simulink model "pressure_tank"  (R2017b)
settings: Solver=FixedStepAuto  StartTime=0.0  StopTime=100  FixedStep=0.01  RelTol=1e-3
libraries: simulink x1
settings Model: Creator=ernst  LastModifiedBy=ernst
settings DataIOCC: SaveFormat=StructureWithTime  SignalLogging=off  DSMLogging=off

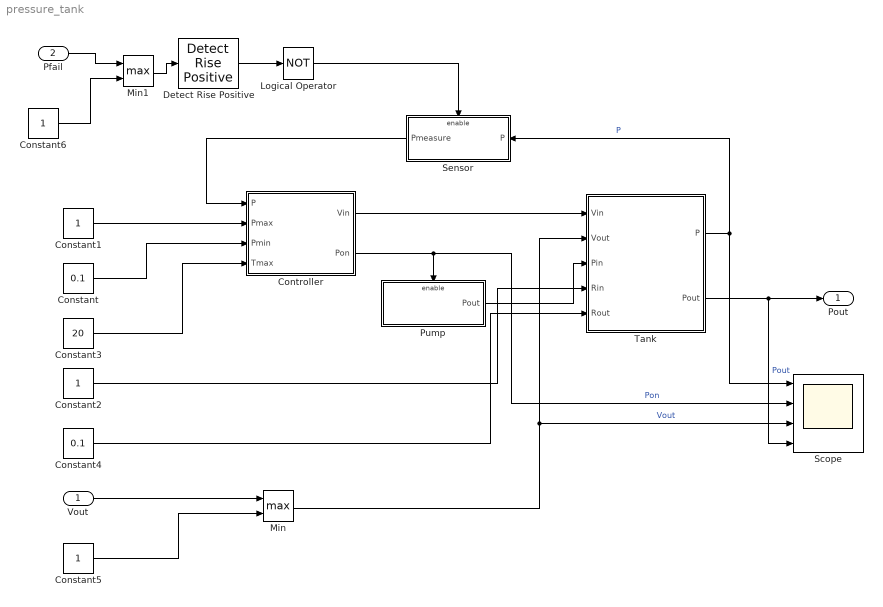
== system pressure_tank ==
  Vout : Inport
  Pfail : Inport  Port=2
  Constant : Constant  Value=0.1
  Constant{1..2,5..6} (4 alike) : Constant
  Constant3 : Constant  Value=20
  Constant4 : Constant  Value=0.1
  Controller : Stateflow chart  TreatAsAtomicUnit=on
  Detect Rise Positive : simulink/Logic and Bit Operations/Detect Rise Positive  vinit=0  OutDataTypeStr=boolean
  Logical Operator : Logic  Operator=NOT  AllPortsSameDT=off  OutDataTypeStr=boolean
  Min : MinMax  Function=max  Inputs=2
  Min1 : MinMax  Function=max  Inputs=2
  Pump : Subsystem
  Scope : Scope  NumInputPorts=4
  Sensor : Subsystem
  Tank : Subsystem
  Pout : Outport
  wires:
  Pump/1(Pout) -> Tank/3(Pin)
  Controller/1(Vin) -> Tank/1(Vin)
  Vout/1 -> Min/1
  Controller/2(Pon) -> Pump/Enable, Scope/2  "Pon"
  Tank/2(Pout) -> Pout/1, Scope/4  "Pout"
  Constant1/1 -> Controller/2(Pmax)
  Constant/1 -> Controller/3(Pmin)
  Tank/1("P ") -> Scope/1, Sensor/1(P)  "P"
  Sensor/1(Pmeasure) -> Controller/1(P)
  Min1/1 -> Detect Rise Positive/1
  Logical Operator/1 -> Sensor/Enable
  Constant2/1 -> Tank/4(Rin)
  Constant3/1 -> Controller/4(Tmax)
  Min/1 -> Tank/2(Vout), Scope/3  "Vout"
  Constant5/1 -> Min/2
  Constant4/1 -> Tank/5(Rout)
  Detect Rise Positive/1 -> Logical Operator/1
  Pfail/1 -> Min1/1
  Constant6/1 -> Min1/2

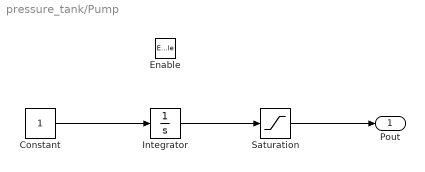
== system pressure_tank/Pump ==
  Enable : EnablePort
  Constant : Constant
  Integrator : Integrator
  Saturation : Saturate  UpperLimit=1  LowerLimit=0
  Pout : Outport
  wires:
  Integrator/1 -> Saturation/1
  Saturation/1 -> Pout/1
  Constant/1 -> Integrator/1

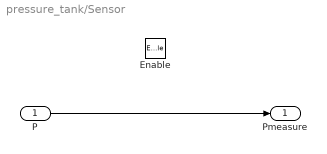
== system pressure_tank/Sensor ==
  P : Inport
  Enable : EnablePort
  Pmeasure : Outport
  wires:
  P/1 -> Pmeasure/1

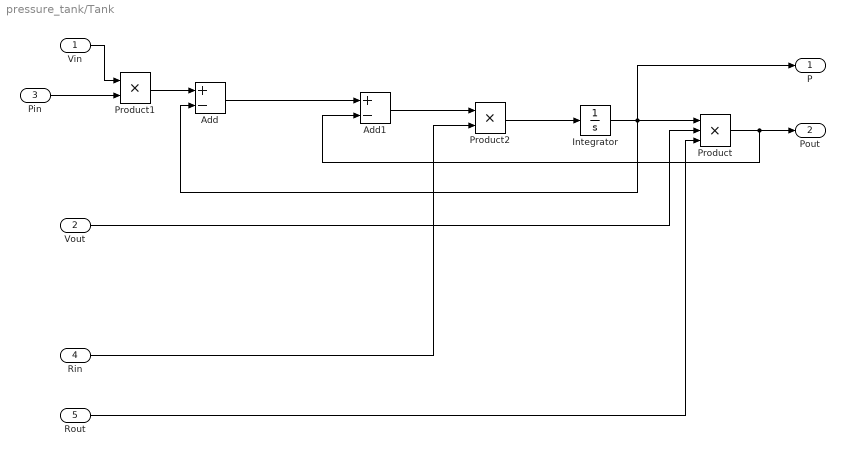
== system pressure_tank/Tank ==
  Vin : Inport
  Vout : Inport  Port=2
  Pin : Inport  Port=3
  Rin : Inport  Port=4
  Rout : Inport  Port=5
  Add : Sum  Inputs=+-
  Add1 : Sum  Inputs=+-
  Integrator : Integrator
  Product : Product  Inputs=3
  Product1 : Product
  Product2 : Product
  "P " : Outport
  Pout : Outport  Port=2
  wires:
  Integrator/1 -> "P "/1, Product/1, Add/2
  Add1/1 -> Product2/1
  Product/1 -> Add1/2, Pout/1
  Product1/1 -> Add/1
  Vin/1 -> Product1/1
  Add/1 -> Add1/1
  Vout/1 -> Product/2
  Pin/1 -> Product1/2
  Product2/1 -> Integrator/1
  Rin/1 -> Product2/2
  Rout/1 -> Product/3

== stateflow chart pressure_tank/Controller ==
  state Idle
    entry:
    Vin = 0;
    Pon = 0;
  state Pumping
    entry:
    Vin = 1;
    Pon = 1;
  (default) -> Idle
  Pumping -> Idle [order 2] : [P >= Pmax]
  Idle -> Pumping : [P <= Pmin]
  Pumping -> Idle [order 1] : after(Tmax,sec)
  data: P input; Pmax input; Pmin input; Vin output; Pon output; Tmax input
